simulink model "CDPM"  (R2013a)
settings: Solver=ode45  StartTime=0.0  StopTime=30  RelTol=1e-3
undefined symbols (not defined in the file): A
libraries: fl_lib x52, dspmtrx3 x21, nesl_utility x16, vrlib x12, simulink x9, elec_lib x8, sdl_lib x4, dspsigops x4, elec_controlled_stepper_lib x4
(part 1 of 2)
settings Model: Creator=Anirudh  LastModifiedBy=Anirudh

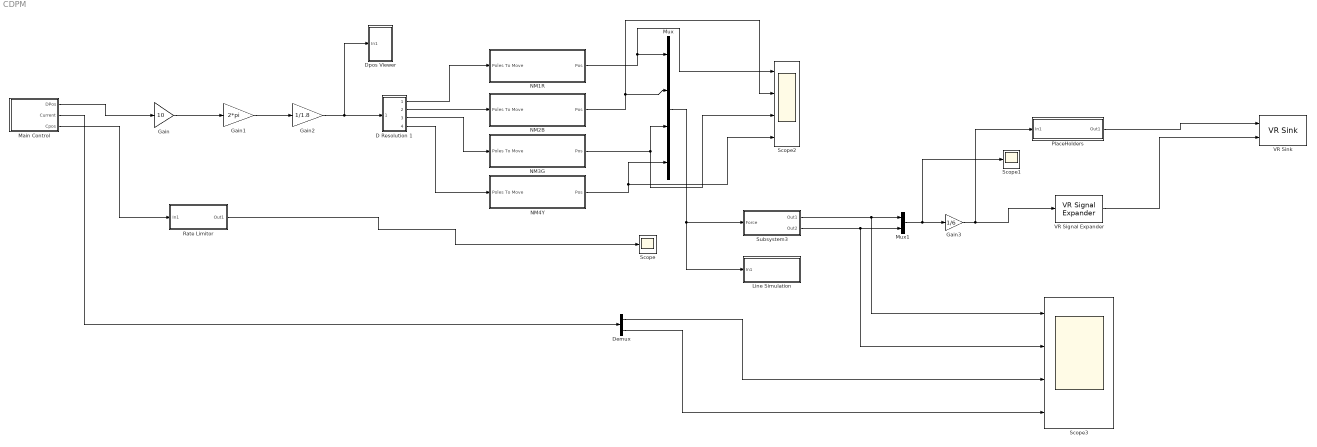
== system CDPM ==
  D Resolution 1 : Subsystem
  Demux : Demux  Outputs=2
  Dpos Viewer : Subsystem
  Gain : Gain  Gain=10
  Gain1 : Gain  Gain=2*pi
  Gain2 : Gain  Gain=1/1.8
  Gain3 : Gain  Gain=1/6
  Line Simulation : Subsystem
  "Main Control " : Subsystem
  Mux : Mux
  Mux1 : Mux  Inputs=2
  "NM1R " : Subsystem
  NM2B : Subsystem
  NM3G : Subsystem
  "NM4Y " : Subsystem
  "PlaceHolders " : Subsystem
  Rate Limitor : Subsystem
  Scope : Scope
      settings: SaveName=ScopeData5
  Scope1 : Scope
      settings: YMin=-3.25  YMax=-1  SaveName=ScopeData7
  Scope2 : Scope  NumInputPorts=4
      settings: TickLabels=on  ShowLegends=on  YMin=-0.79~0.2225~0.309~0.7675  YMax=-0.7675~0.24~0.318~0.79
  Scope3 : Scope  NumInputPorts=4
      settings: YMin=-5~-5~-5~-5  YMax=5~5~5~5  SaveName=ScopeData8
  Subsystem3 : Subsystem
  VR Signal Expander : vrlib/VR Signal Expander  outwidth=3  outidx=[1 3]
  VR Sink : vrlib/VR Sink  InstantiateOnLoad=on  SampleTime=0.1  ViewEnable=on  RemoteChange=off  RemoteView=off  FieldsWritten=LINES.point.3.-1.1.double#EoF.translation.3.1.1.double  WorldFileName=CDPM.wrl  AutoView=on  VideoDimensions=[]  AllowVariableSize=off
  wires:
  "Main Control "/1("DPos ") -> Gain/1
  Gain/1 -> Gain1/1
  Gain1/1 -> Gain2/1
  Gain2/1 -> D Resolution 1/1(In1), Dpos Viewer/1(In1)
  D Resolution 1/1(Out1) -> "NM1R "/1("Poles To Move ")
  "Main Control "/2("Current ") -> Demux/1
  "NM1R "/1(Pos) -> Scope2/1, Mux/1
  D Resolution 1/2(Out2) -> NM2B/1("Poles To Move ")
  D Resolution 1/3(Out3) -> NM3G/1("Poles To Move ")
  D Resolution 1/4(Out4) -> "NM4Y "/1("Poles To Move ")
  "NM4Y "/1(Pos) -> Mux/4, Scope2/4
  NM2B/1(Pos) -> Scope2/2, Mux/2
  NM3G/1(Pos) -> Mux/3, Scope2/3
  Subsystem3/1(Out1) -> Scope3/1, Mux1/1
  Subsystem3/2(Out2) -> Scope3/2, Mux1/2
  "Main Control "/3(Cpos) -> Rate Limitor/1(In1)
  Rate Limitor/1(Out1) -> Scope/1
  Mux1/1 -> Scope1/1, Gain3/1
  Gain3/1 -> "PlaceHolders "/1(In1), VR Signal Expander/1
  Demux/1 -> Scope3/3
  Demux/2 -> Scope3/4
  VR Signal Expander/1 -> VR Sink/2
  "PlaceHolders "/1(Out1) -> VR Sink/1
  Mux/1 -> Line Simulation/1(In1), Subsystem3/1(Force)

== system CDPM/D Resolution 1 ==
  In1 : Inport
  Submatrix : dspmtrx3/Submatrix  RowSpan=All rows  RowStartMode=First  RowStartIndex=1  RowEndMode=Last  RowEndIndex=1  ColSpan=One column  ColStartMode=Index  ColStartIndex=1  ColEndMode=Last  ColEndIndex=1
  Submatrix1 : dspmtrx3/Submatrix  RowSpan=One row  RowStartMode=Index  RowStartIndex=1  RowEndMode=Last  RowEndIndex=1  ColSpan=One column  ColStartMode=Index  ColStartIndex=2  ColEndMode=Last  ColEndIndex=1
  Submatrix2 : dspmtrx3/Submatrix  RowSpan=All rows  RowStartMode=Index  RowStartIndex=2  RowEndMode=Last  RowEndIndex=1  ColSpan=One column  ColStartMode=Index  ColStartIndex=3  ColEndMode=Last  ColEndIndex=1
  Submatrix3 : dspmtrx3/Submatrix  RowSpan=All rows  RowStartMode=Index  RowStartIndex=2  RowEndMode=Last  RowEndIndex=1  ColSpan=One column  ColStartMode=Index  ColStartIndex=4  ColEndMode=Last  ColEndIndex=1
  Out1 : Outport
  Out2 : Outport  Port=2
  Out3 : Outport  Port=3
  Out4 : Outport  Port=4
  wires:
  Submatrix2/1 -> Out3/1
  Submatrix1/1 -> Out2/1
  Submatrix3/1 -> Out4/1
  Submatrix/1 -> Out1/1
  In1/1 -> Submatrix/1, Submatrix1/1, Submatrix2/1, Submatrix3/1

== system CDPM/Dpos Viewer ==
  In1 : Inport
  D Resolution 1 : Subsystem
  Scope1 : Scope  NumInputPorts=4
      settings: TimeRange=5  YMin=-700~-800~-300~-200  YMax=400~700~700~400  SaveName=ScopeData3
  wires:
  D Resolution 1/4(Out4) -> Scope1/4
  D Resolution 1/2(Out2) -> Scope1/2
  D Resolution 1/1(Out1) -> Scope1/1
  In1/1 -> D Resolution 1/1(In1)
  D Resolution 1/3(Out3) -> Scope1/3

== system CDPM/Line Simulation ==
  In1 : Inport
  Demux : Demux
  VR Signal Expander{,1..3} (4 alike) : vrlib/VR Signal Expander  outwidth=4  outidx=[4]
  VR Sink : vrlib/VR Sink  InstantiateOnLoad=on  SampleTime=0.1  ViewEnable=on  RemoteChange=off  RemoteView=off  FieldsWritten=N2YR.rotation.4.1.1.double#N1RR.rotation.4.1.1.double#N3BR.rotation.4.1.1.double#N4GR.rotation.4.1.1.double  WorldFileName=CDPM.wrl  AutoView=off  VideoDimensions=[]  AllowVariableSize=off
  wires:
  VR Signal Expander/1 -> VR Sink/2
  In1/1 -> Demux/1
  Demux/1 -> VR Signal Expander/1
  Demux/2 -> VR Signal Expander1/1
  VR Signal Expander2/1 -> VR Sink/3
  Demux/3 -> VR Signal Expander2/1
  VR Signal Expander3/1 -> VR Sink/4
  Demux/4 -> VR Signal Expander3/1
  VR Signal Expander1/1 -> VR Sink/1

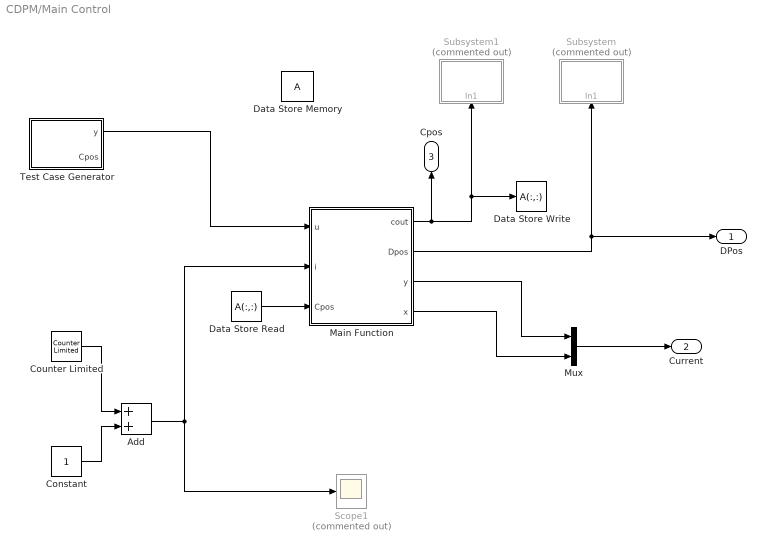
== system CDPM/Main Control  ==
  Add : Sum
  Constant : Constant
  Counter Limited : simulink/Sources/Counter Limited  uplimit=15  tsamp=1
  Data Store Memory : DataStoreMemory  ReadBeforeWriteMsg=warning  WriteAfterWriteMsg=warning  WriteAfterReadMsg=warning  InitialValue=[30,30,30,30]  VectorParams1D=off
  Data Store Read : DataStoreRead  SampleTime=1  DataStoreElements=A(:,:)
  Data Store Write : DataStoreWrite  SampleTime=2  DataStoreElements=A(:,:)
  "Main Function " : MATLAB Function  TreatAsAtomicUnit=on  SystemSampleTime=1
  Mux : Mux  Inputs=2
  Scope1 : Scope  Commented=on
      settings: SaveName=ScopeData6
  Subsystem : Subsystem  Commented=on
  Subsystem1 : Subsystem  Commented=on
  "Test Case Generator " : MATLAB Function
  "DPos " : Outport
  "Current " : Outport  Port=2
  Cpos : Outport  Port=3
  wires:
  Constant/1 -> Add/2
  "Main Function "/2(Dpos) -> "DPos "/1, Subsystem/1(In1)
  Counter Limited/1 -> Add/1
  Add/1 -> "Main Function "/2(i), Scope1/1
  "Main Function "/1(cout) -> Subsystem1/1(In1), Data Store Write/1, Cpos/1
  "Test Case Generator "/1(y) -> "Main Function "/1(u)
  Mux/1 -> "Current "/1
  "Main Function "/3(y) -> Mux/1
  "Main Function "/4(x) -> Mux/2
  Data Store Read/1 -> "Main Function "/3(Cpos)

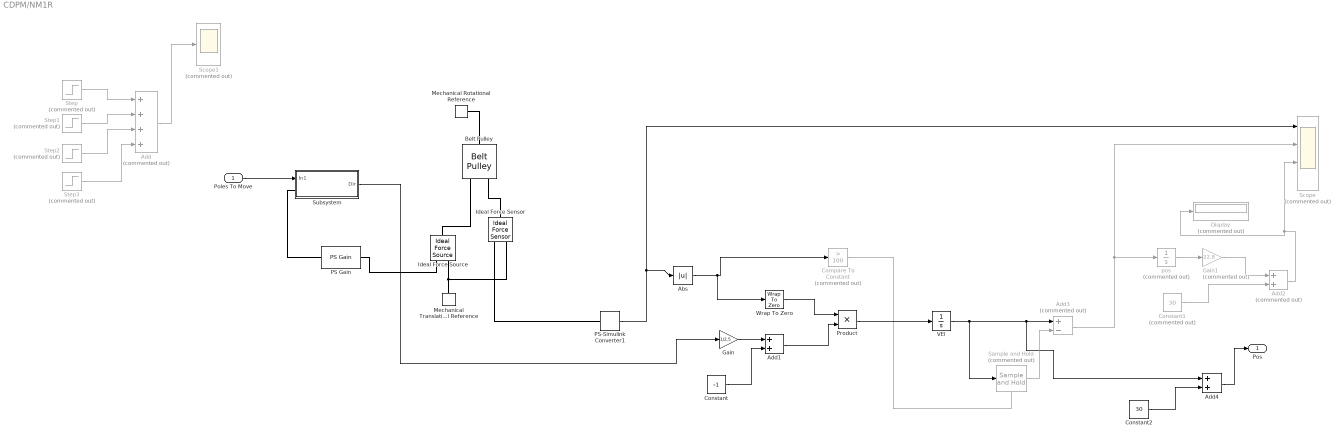
== system CDPM/NM1R  ==
  "Poles To Move " : Inport
  Abs : Abs
  Add : Sum  Commented=on  Inputs=++++
  Add1 : Sum
  Add2 : Sum  Commented=on
  Add3 : Sum  Commented=on  Inputs=+-
  Add4 : Sum
  Belt Pulley : sdl_lib/Couplings & Drives/Belt Pulley  belt_type=1  sheave_ang=30 deg  num_belts=1  linear_density=0.6 kg/m  breakable=0  F_max=1e+5 N  check_tension=0  r_pulley=0.15 m  b_pulley=0.001 N*m/(rad/s)  model_inertia=0  pulley_inertia=0.01 kg*m^2  initial_velocity=0 rad/s  mu=0.5  phi_wrap=180 deg  v_thr=0.001 m/s  LocalVarLogging=[]
  Compare To Constant : simulink/Logic and Bit Operations/Compare To Constant  Commented=on  relop=>  const=100  OutDataTypeStr=uint8
  Constant : Constant  Value=-1
  Constant1 : Constant  Commented=on  Value=30
  Constant2 : Constant  Value=30
  Display : Display  Commented=on
  Gain : Gain  Gain=1/2.5
  Gain1 : Gain  Commented=on  Gain=22.8
  Ideal Force Sensor : fl_lib/Mechanical/Mechanical Sensors/Ideal Force Sensor  v_Log=off  f_Log=off  LocalVarNames=|v|f  LocalVarDescs=|v|f  LocalVarLogging=[0 0]
  Ideal Force Source : fl_lib/Mechanical/Mechanical Sources/Ideal Force Source  v_Log=off  f_Log=off  LocalVarNames=|v|f  LocalVarDescs=|v|f  LocalVarLogging=[0 0]
  Mechanical Rotational Reference : fl_lib/Mechanical/Rotational Elements/Mechanical Rotational Reference  t_Log=off  LocalVarNames=|t  LocalVarDescs=|t  LocalVarLogging=0
  Mechanical Translational Reference : fl_lib/Mechanical/Translational Elements/Mechanical Translational Reference  f_Log=off  LocalVarNames=|f  LocalVarDescs=|f  LocalVarLogging=0
  PS Gain : fl_lib/Physical Signals/Functions/PS Gain  gain=100  LocalVarLogging=[]
  PS-Simulink Converter1 : nesl_utility/PS-Simulink Converter  PhysicalDomain=network_engine_domain  SubClassName=ps_output  LeftPortType=input  RightPortType=output  PseudoPeriodic=off  Frequencies=[]  Unit=N  AffineConversion=off
  Product : Product
  Sample and Hold : dspsigops/Sample and Hold  Commented=on  trig=Either edge  initCond=0  latchinput=off
  Scope : Scope  Commented=on  NumInputPorts=4
      settings: TickLabels=on  YMin=-5~-5~-5~-5  YMax=5~5~5~5  SaveName=ScopeData4
  Scope1 : Scope  Commented=on
  Step : Step  Commented=on  Time=5  After=10  SampleTime=0
  Step1 : Step  Commented=on  Time=10  After=10  SampleTime=0
  Step2 : Step  Commented=on  Time=15  After=-10  SampleTime=0
  Step3 : Step  Commented=on  Time=20  After=-10  SampleTime=0
  Subsystem : Subsystem
  VEl : Integrator
  Wrap To Zero : simulink/Discontinuities/Wrap To Zero  Threshold=50
  pos : Integrator  Commented=on
  Pos : Outport
  wires:
  Add/1 -> Scope1/1
  Step/1 -> Add/1
  Step1/1 -> Add/2
  Step2/1 -> Add/3
  Step3/1 -> Add/4
  "Poles To Move "/1 -> Subsystem/1(In1)
  Subsystem/1("Dir ") -> Gain/1
  Gain/1 -> Add1/1
  Constant/1 -> Add1/2
  Add1/1 -> Product/2
  Abs/1 -> Wrap To Zero/1, Compare To Constant/1
  Constant1/1 -> Add2/2
  pos/1 -> Gain1/1
  Gain1/1 -> Add2/1
  VEl/1 -> Sample and Hold/1, Add4/1, Add3/1
  Sample and Hold/1 -> Add3/2
  Add3/1 -> pos/1, Scope/2
  Add2/1 -> Scope/3, Display/1
  PS-Simulink Converter1/1 -> Scope/1, Abs/1
  Compare To Constant/1 -> Sample and Hold/Trigger
  Wrap To Zero/1 -> Product/1
  Constant2/1 -> Add4/2
  Add4/1 -> Pos/1
  Product/1 -> VEl/1
  connections:
  Ideal Force Source/RConn2 -- Ideal Force Sensor/RConn1 -- Mechanical Translational Reference/LConn1
  PS Gain/RConn1 -- Ideal Force Source/RConn1
  Belt Pulley/RConn2 -- Ideal Force Source/LConn1
  Subsystem/LConn1 -- PS Gain/LConn1
  Belt Pulley/RConn1 -- Ideal Force Sensor/LConn1
  PS-Simulink Converter1/LConn1 -- Ideal Force Sensor/RConn2
  Mechanical Rotational Reference/LConn1 -- Belt Pulley/LConn1

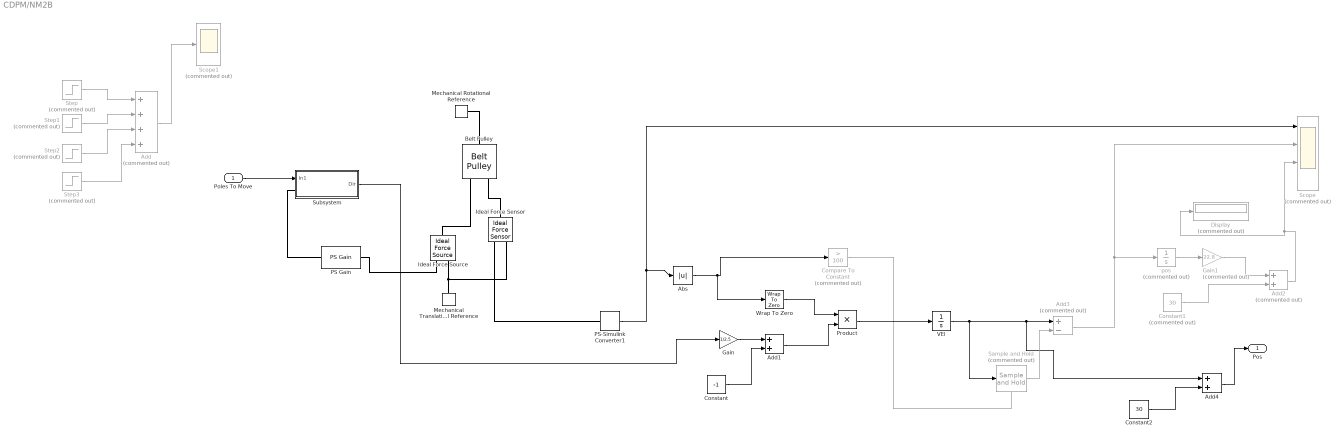
== system CDPM/NM2B ==
  "Poles To Move " : Inport
  Abs : Abs
  Add : Sum  Commented=on  Inputs=++++
  Add1 : Sum
  Add2 : Sum  Commented=on
  Add3 : Sum  Commented=on  Inputs=+-
  Add4 : Sum
  Belt Pulley : sdl_lib/Couplings & Drives/Belt Pulley  belt_type=1  sheave_ang=30 deg  num_belts=1  linear_density=0.6 kg/m  breakable=0  F_max=1e+5 N  check_tension=0  r_pulley=0.15 m  b_pulley=0.001 N*m/(rad/s)  model_inertia=0  pulley_inertia=0.01 kg*m^2  initial_velocity=0 rad/s  mu=0.5  phi_wrap=180 deg  v_thr=0.001 m/s  LocalVarLogging=[]
  Compare To Constant : simulink/Logic and Bit Operations/Compare To Constant  Commented=on  relop=>  const=100  OutDataTypeStr=uint8
  Constant : Constant  Value=-1
  Constant1 : Constant  Commented=on  Value=30
  Constant2 : Constant  Value=30
  Display : Display  Commented=on
  Gain : Gain  Gain=1/2.5
  Gain1 : Gain  Commented=on  Gain=22.8
  Ideal Force Sensor : fl_lib/Mechanical/Mechanical Sensors/Ideal Force Sensor  v_Log=off  f_Log=off  LocalVarNames=|v|f  LocalVarDescs=|v|f  LocalVarLogging=[0 0]
  Ideal Force Source : fl_lib/Mechanical/Mechanical Sources/Ideal Force Source  v_Log=off  f_Log=off  LocalVarNames=|v|f  LocalVarDescs=|v|f  LocalVarLogging=[0 0]
  Mechanical Rotational Reference : fl_lib/Mechanical/Rotational Elements/Mechanical Rotational Reference  t_Log=off  LocalVarNames=|t  LocalVarDescs=|t  LocalVarLogging=0
  Mechanical Translational Reference : fl_lib/Mechanical/Translational Elements/Mechanical Translational Reference  f_Log=off  LocalVarNames=|f  LocalVarDescs=|f  LocalVarLogging=0
  PS Gain : fl_lib/Physical Signals/Functions/PS Gain  gain=100  LocalVarLogging=[]
  PS-Simulink Converter1 : nesl_utility/PS-Simulink Converter  PhysicalDomain=network_engine_domain  SubClassName=ps_output  LeftPortType=input  RightPortType=output  PseudoPeriodic=off  Frequencies=[]  Unit=N  AffineConversion=off
  Product : Product
  Sample and Hold : dspsigops/Sample and Hold  Commented=on  trig=Either edge  initCond=0  latchinput=off
  Scope : Scope  Commented=on  NumInputPorts=4
      settings: TickLabels=on  YMin=-5~-5~-5~-5  YMax=5~5~5~5  SaveName=ScopeData4
  Scope1 : Scope  Commented=on
  Step : Step  Commented=on  Time=5  After=10  SampleTime=0
  Step1 : Step  Commented=on  Time=10  After=10  SampleTime=0
  Step2 : Step  Commented=on  Time=15  After=-10  SampleTime=0
  Step3 : Step  Commented=on  Time=20  After=-10  SampleTime=0
  Subsystem : Subsystem
  VEl : Integrator
  Wrap To Zero : simulink/Discontinuities/Wrap To Zero  Threshold=50
  pos : Integrator  Commented=on
  Pos : Outport
  wires:
  Add/1 -> Scope1/1
  Step/1 -> Add/1
  Step1/1 -> Add/2
  Step2/1 -> Add/3
  Step3/1 -> Add/4
  "Poles To Move "/1 -> Subsystem/1(In1)
  Subsystem/1("Dir ") -> Gain/1
  Gain/1 -> Add1/1
  Constant/1 -> Add1/2
  Add1/1 -> Product/2
  Abs/1 -> Wrap To Zero/1, Compare To Constant/1
  Constant1/1 -> Add2/2
  pos/1 -> Gain1/1
  Gain1/1 -> Add2/1
  VEl/1 -> Sample and Hold/1, Add4/1, Add3/1
  Sample and Hold/1 -> Add3/2
  Add3/1 -> pos/1, Scope/2
  Add2/1 -> Scope/3, Display/1
  PS-Simulink Converter1/1 -> Scope/1, Abs/1
  Compare To Constant/1 -> Sample and Hold/Trigger
  Wrap To Zero/1 -> Product/1
  Constant2/1 -> Add4/2
  Add4/1 -> Pos/1
  Product/1 -> VEl/1
  connections:
  Ideal Force Source/RConn2 -- Ideal Force Sensor/RConn1 -- Mechanical Translational Reference/LConn1
  PS Gain/RConn1 -- Ideal Force Source/RConn1
  Belt Pulley/RConn2 -- Ideal Force Source/LConn1
  Subsystem/LConn1 -- PS Gain/LConn1
  Belt Pulley/RConn1 -- Ideal Force Sensor/LConn1
  PS-Simulink Converter1/LConn1 -- Ideal Force Sensor/RConn2
  Mechanical Rotational Reference/LConn1 -- Belt Pulley/LConn1

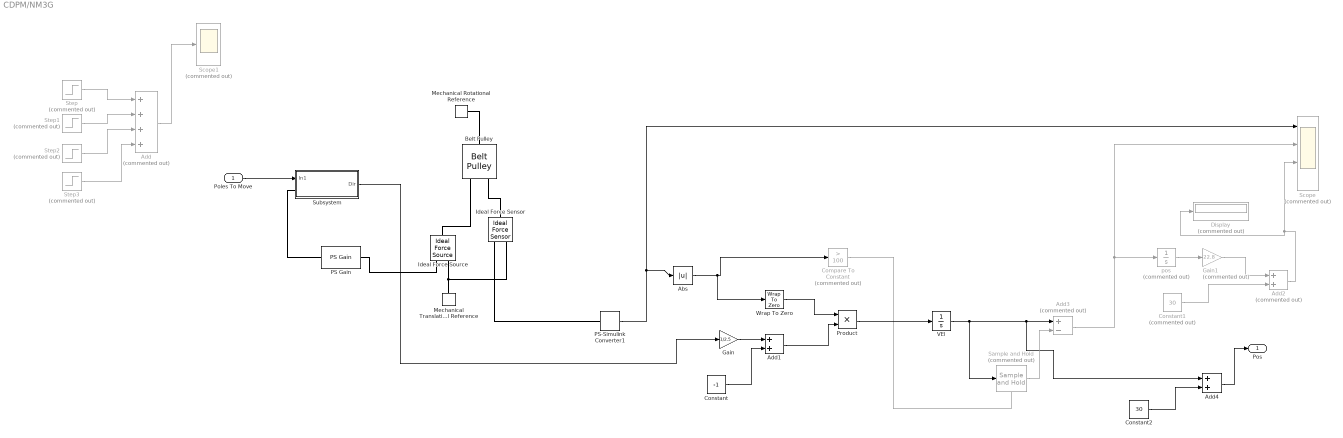
== system CDPM/NM3G ==
  "Poles To Move " : Inport
  Abs : Abs
  Add : Sum  Commented=on  Inputs=++++
  Add1 : Sum
  Add2 : Sum  Commented=on
  Add3 : Sum  Commented=on  Inputs=+-
  Add4 : Sum
  Belt Pulley : sdl_lib/Couplings & Drives/Belt Pulley  belt_type=1  sheave_ang=30 deg  num_belts=1  linear_density=0.6 kg/m  breakable=0  F_max=1e+5 N  check_tension=0  r_pulley=0.15 m  b_pulley=0.001 N*m/(rad/s)  model_inertia=0  pulley_inertia=0.01 kg*m^2  initial_velocity=0 rad/s  mu=0.5  phi_wrap=180 deg  v_thr=0.001 m/s  LocalVarLogging=[]
  Compare To Constant : simulink/Logic and Bit Operations/Compare To Constant  Commented=on  relop=>  const=100  OutDataTypeStr=uint8
  Constant : Constant  Value=-1
  Constant1 : Constant  Commented=on  Value=30
  Constant2 : Constant  Value=30
  Display : Display  Commented=on
  Gain : Gain  Gain=1/2.5
  Gain1 : Gain  Commented=on  Gain=22.8
  Ideal Force Sensor : fl_lib/Mechanical/Mechanical Sensors/Ideal Force Sensor  v_Log=off  f_Log=off  LocalVarNames=|v|f  LocalVarDescs=|v|f  LocalVarLogging=[0 0]
  Ideal Force Source : fl_lib/Mechanical/Mechanical Sources/Ideal Force Source  v_Log=off  f_Log=off  LocalVarNames=|v|f  LocalVarDescs=|v|f  LocalVarLogging=[0 0]
  Mechanical Rotational Reference : fl_lib/Mechanical/Rotational Elements/Mechanical Rotational Reference  t_Log=off  LocalVarNames=|t  LocalVarDescs=|t  LocalVarLogging=0
  Mechanical Translational Reference : fl_lib/Mechanical/Translational Elements/Mechanical Translational Reference  f_Log=off  LocalVarNames=|f  LocalVarDescs=|f  LocalVarLogging=0
  PS Gain : fl_lib/Physical Signals/Functions/PS Gain  gain=100  LocalVarLogging=[]
  PS-Simulink Converter1 : nesl_utility/PS-Simulink Converter  PhysicalDomain=network_engine_domain  SubClassName=ps_output  LeftPortType=input  RightPortType=output  PseudoPeriodic=off  Frequencies=[]  Unit=N  AffineConversion=off
  Product : Product
  Sample and Hold : dspsigops/Sample and Hold  Commented=on  trig=Either edge  initCond=0  latchinput=off
  Scope : Scope  Commented=on  NumInputPorts=4
      settings: TickLabels=on  YMin=-5~-5~-5~-5  YMax=5~5~5~5  SaveName=ScopeData4
  Scope1 : Scope  Commented=on
  Step : Step  Commented=on  Time=5  After=10  SampleTime=0
  Step1 : Step  Commented=on  Time=10  After=10  SampleTime=0
  Step2 : Step  Commented=on  Time=15  After=-10  SampleTime=0
  Step3 : Step  Commented=on  Time=20  After=-10  SampleTime=0
  Subsystem : Subsystem
  VEl : Integrator
  Wrap To Zero : simulink/Discontinuities/Wrap To Zero  Threshold=50
  pos : Integrator  Commented=on
  Pos : Outport
  wires:
  Add/1 -> Scope1/1
  Step/1 -> Add/1
  Step1/1 -> Add/2
  Step2/1 -> Add/3
  Step3/1 -> Add/4
  "Poles To Move "/1 -> Subsystem/1(In1)
  Subsystem/1("Dir ") -> Gain/1
  Gain/1 -> Add1/1
  Constant/1 -> Add1/2
  Add1/1 -> Product/2
  Abs/1 -> Wrap To Zero/1, Compare To Constant/1
  Constant1/1 -> Add2/2
  pos/1 -> Gain1/1
  Gain1/1 -> Add2/1
  VEl/1 -> Sample and Hold/1, Add4/1, Add3/1
  Sample and Hold/1 -> Add3/2
  Add3/1 -> pos/1, Scope/2
  Add2/1 -> Scope/3, Display/1
  PS-Simulink Converter1/1 -> Scope/1, Abs/1
  Compare To Constant/1 -> Sample and Hold/Trigger
  Wrap To Zero/1 -> Product/1
  Constant2/1 -> Add4/2
  Add4/1 -> Pos/1
  Product/1 -> VEl/1
  connections:
  Ideal Force Source/RConn2 -- Ideal Force Sensor/RConn1 -- Mechanical Translational Reference/LConn1
  PS Gain/RConn1 -- Ideal Force Source/RConn1
  Belt Pulley/RConn2 -- Ideal Force Source/LConn1
  Subsystem/LConn1 -- PS Gain/LConn1
  Belt Pulley/RConn1 -- Ideal Force Sensor/LConn1
  PS-Simulink Converter1/LConn1 -- Ideal Force Sensor/RConn2
  Mechanical Rotational Reference/LConn1 -- Belt Pulley/LConn1

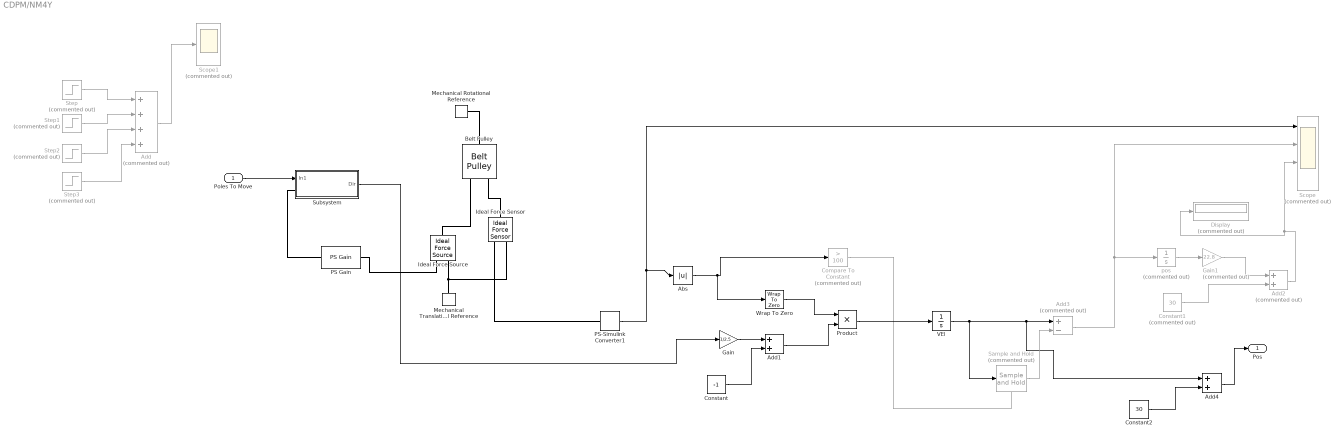
== system CDPM/NM4Y  ==
  "Poles To Move " : Inport
  Abs : Abs
  Add : Sum  Commented=on  Inputs=++++
  Add1 : Sum
  Add2 : Sum  Commented=on
  Add3 : Sum  Commented=on  Inputs=+-
  Add4 : Sum
  Belt Pulley : sdl_lib/Couplings & Drives/Belt Pulley  belt_type=1  sheave_ang=30 deg  num_belts=1  linear_density=0.6 kg/m  breakable=0  F_max=1e+5 N  check_tension=0  r_pulley=0.15 m  b_pulley=0.001 N*m/(rad/s)  model_inertia=0  pulley_inertia=0.01 kg*m^2  initial_velocity=0 rad/s  mu=0.5  phi_wrap=180 deg  v_thr=0.001 m/s  LocalVarLogging=[]
  Compare To Constant : simulink/Logic and Bit Operations/Compare To Constant  Commented=on  relop=>  const=100  OutDataTypeStr=uint8
  Constant : Constant  Value=-1
  Constant1 : Constant  Commented=on  Value=30
  Constant2 : Constant  Value=30
  Display : Display  Commented=on
  Gain : Gain  Gain=1/2.5
  Gain1 : Gain  Commented=on  Gain=22.8
  Ideal Force Sensor : fl_lib/Mechanical/Mechanical Sensors/Ideal Force Sensor  v_Log=off  f_Log=off  LocalVarNames=|v|f  LocalVarDescs=|v|f  LocalVarLogging=[0 0]
  Ideal Force Source : fl_lib/Mechanical/Mechanical Sources/Ideal Force Source  v_Log=off  f_Log=off  LocalVarNames=|v|f  LocalVarDescs=|v|f  LocalVarLogging=[0 0]
  Mechanical Rotational Reference : fl_lib/Mechanical/Rotational Elements/Mechanical Rotational Reference  t_Log=off  LocalVarNames=|t  LocalVarDescs=|t  LocalVarLogging=0
  Mechanical Translational Reference : fl_lib/Mechanical/Translational Elements/Mechanical Translational Reference  f_Log=off  LocalVarNames=|f  LocalVarDescs=|f  LocalVarLogging=0
  PS Gain : fl_lib/Physical Signals/Functions/PS Gain  gain=100  LocalVarLogging=[]
  PS-Simulink Converter1 : nesl_utility/PS-Simulink Converter  PhysicalDomain=network_engine_domain  SubClassName=ps_output  LeftPortType=input  RightPortType=output  PseudoPeriodic=off  Frequencies=[]  Unit=N  AffineConversion=off
  Product : Product
  Sample and Hold : dspsigops/Sample and Hold  Commented=on  trig=Either edge  initCond=0  latchinput=off
  Scope : Scope  Commented=on  NumInputPorts=4
      settings: TickLabels=on  YMin=-5~-5~-5~-5  YMax=5~5~5~5  SaveName=ScopeData4
  Scope1 : Scope  Commented=on
  Step : Step  Commented=on  Time=5  After=10  SampleTime=0
  Step1 : Step  Commented=on  Time=10  After=10  SampleTime=0
  Step2 : Step  Commented=on  Time=15  After=-10  SampleTime=0
  Step3 : Step  Commented=on  Time=20  After=-10  SampleTime=0
  Subsystem : Subsystem
  VEl : Integrator
  Wrap To Zero : simulink/Discontinuities/Wrap To Zero  Threshold=50
  pos : Integrator  Commented=on
  Pos : Outport
  wires:
  Add/1 -> Scope1/1
  Step/1 -> Add/1
  Step1/1 -> Add/2
  Step2/1 -> Add/3
  Step3/1 -> Add/4
  "Poles To Move "/1 -> Subsystem/1(In1)
  Subsystem/1("Dir ") -> Gain/1
  Gain/1 -> Add1/1
  Constant/1 -> Add1/2
  Add1/1 -> Product/2
  Abs/1 -> Wrap To Zero/1, Compare To Constant/1
  Constant1/1 -> Add2/2
  pos/1 -> Gain1/1
  Gain1/1 -> Add2/1
  VEl/1 -> Sample and Hold/1, Add4/1, Add3/1
  Sample and Hold/1 -> Add3/2
  Add3/1 -> pos/1, Scope/2
  Add2/1 -> Scope/3, Display/1
  PS-Simulink Converter1/1 -> Scope/1, Abs/1
  Compare To Constant/1 -> Sample and Hold/Trigger
  Wrap To Zero/1 -> Product/1
  Constant2/1 -> Add4/2
  Add4/1 -> Pos/1
  Product/1 -> VEl/1
  connections:
  Ideal Force Source/RConn2 -- Ideal Force Sensor/RConn1 -- Mechanical Translational Reference/LConn1
  PS Gain/RConn1 -- Ideal Force Source/RConn1
  Belt Pulley/RConn2 -- Ideal Force Source/LConn1
  Subsystem/LConn1 -- PS Gain/LConn1
  Belt Pulley/RConn1 -- Ideal Force Sensor/LConn1
  PS-Simulink Converter1/LConn1 -- Ideal Force Sensor/RConn2
  Mechanical Rotational Reference/LConn1 -- Belt Pulley/LConn1

== system CDPM/PlaceHolders  ==
  In1 : Inport
  Matrix Concatenate : Concatenate  NumInputs=5  Mode=Multidimensional array
  Transpose{,1..4} (5 alike) : dspmtrx3/Transpose  Hermitian=off  overflowFlag=off
  VR Placeholder{,1..3} (4 alike) : vrlib/VR Placeholder  outwidth=3
  VR Signal Expander1 : vrlib/VR Signal Expander  outwidth=3  outidx=[1 3]
  Out1 : Outport
  wires:
  VR Placeholder2/1 -> Transpose3/1
  Transpose3/1 -> Matrix Concatenate/4
  Transpose1/1 -> Matrix Concatenate/2
  Transpose2/1 -> Matrix Concatenate/3
  Matrix Concatenate/1 -> Out1/1
  Transpose4/1 -> Matrix Concatenate/5
  VR Placeholder/1 -> Transpose1/1
  VR Placeholder3/1 -> Transpose4/1
  VR Signal Expander1/1 -> Transpose/1
  VR Placeholder1/1 -> Transpose2/1
  Transpose/1 -> Matrix Concatenate/1
  In1/1 -> VR Signal Expander1/1

== system CDPM/Rate Limitor ==
  In1 : Inport
  Demux : Demux
  Mux : Mux
  Rate Limiter{,1..3} (4 alike) : RateLimiter  RisingSlewLimit=25  FallingSlewLimit=-25
  Out1 : Outport
  wires:
  In1/1 -> Demux/1
  Demux/1 -> Rate Limiter/1
  Demux/2 -> Rate Limiter1/1
  Demux/3 -> Rate Limiter2/1
  Demux/4 -> Rate Limiter3/1
  Rate Limiter3/1 -> Mux/4
  Rate Limiter/1 -> Mux/1
  Rate Limiter2/1 -> Mux/3
  Rate Limiter1/1 -> Mux/2
  Mux/1 -> Out1/1

== system CDPM/Subsystem3 ==
  Force : Inport
  Constant : Constant  Value=40
  Demux1 : Demux
  Herons Formula : Subsystem
  Herons Formula1 : Subsystem
  Out1 : Outport
  Out2 : Outport  Port=2
  wires:
  Force/1 -> Demux1/1
  Demux1/1 -> Herons Formula/1(In1)
  Demux1/2 -> Herons Formula1/1(In1), Herons Formula/2(In2)
  Constant/1 -> Herons Formula/3(In3), Herons Formula1/3(In3)
  Herons Formula/1(Out1) -> Out1/1
  Herons Formula1/1(Out1) -> Out2/1
  Demux1/4 -> Herons Formula1/2(In2)

== system CDPM/Dpos Viewer/D Resolution 1 ==
  In1 : Inport
  Submatrix : dspmtrx3/Submatrix  RowSpan=All rows  RowStartMode=First  RowStartIndex=1  RowEndMode=Last  RowEndIndex=1  ColSpan=One column  ColStartMode=Index  ColStartIndex=1  ColEndMode=Last  ColEndIndex=1
  Submatrix1 : dspmtrx3/Submatrix  RowSpan=One row  RowStartMode=Index  RowStartIndex=1  RowEndMode=Last  RowEndIndex=1  ColSpan=One column  ColStartMode=Index  ColStartIndex=2  ColEndMode=Last  ColEndIndex=1
  Submatrix2 : dspmtrx3/Submatrix  RowSpan=All rows  RowStartMode=Index  RowStartIndex=2  RowEndMode=Last  RowEndIndex=1  ColSpan=One column  ColStartMode=Index  ColStartIndex=3  ColEndMode=Last  ColEndIndex=1
  Submatrix3 : dspmtrx3/Submatrix  RowSpan=All rows  RowStartMode=Index  RowStartIndex=2  RowEndMode=Last  RowEndIndex=1  ColSpan=One column  ColStartMode=Index  ColStartIndex=4  ColEndMode=Last  ColEndIndex=1
  Out1 : Outport
  Out2 : Outport  Port=2
  Out3 : Outport  Port=3
  Out4 : Outport  Port=4
  wires:
  Submatrix2/1 -> Out3/1
  Submatrix1/1 -> Out2/1
  Submatrix3/1 -> Out4/1
  Submatrix/1 -> Out1/1
  In1/1 -> Submatrix/1, Submatrix1/1, Submatrix2/1, Submatrix3/1

== system CDPM/Main Control /Subsystem ==
  In1 : Inport
  "D Resolution " : Subsystem
  Scope : Scope  NumInputPorts=4
      settings: YMin=-5~-5~-5~-5  YMax=5~5~5~5  SaveName=ScopeData2
  wires:
  In1/1 -> "D Resolution "/1(In1)
  "D Resolution "/3(Out3) -> Scope/3
  "D Resolution "/2(Out2) -> Scope/2
  "D Resolution "/4(Out4) -> Scope/4
  "D Resolution "/1(Out1) -> Scope/1

== system CDPM/Main Control /Subsystem1 ==
  In1 : Inport
  D Resolution 1 : Subsystem
  Display : Display
  Scope1 : Scope  NumInputPorts=4
      settings: YMin=-5~-5~-5~-5  YMax=5~5~5~5  SaveName=ScopeData3
  wires:
  D Resolution 1/4(Out4) -> Scope1/4
  D Resolution 1/2(Out2) -> Scope1/2
  D Resolution 1/1(Out1) -> Display/1, Scope1/1
  In1/1 -> D Resolution 1/1(In1)
  D Resolution 1/3(Out3) -> Scope1/3

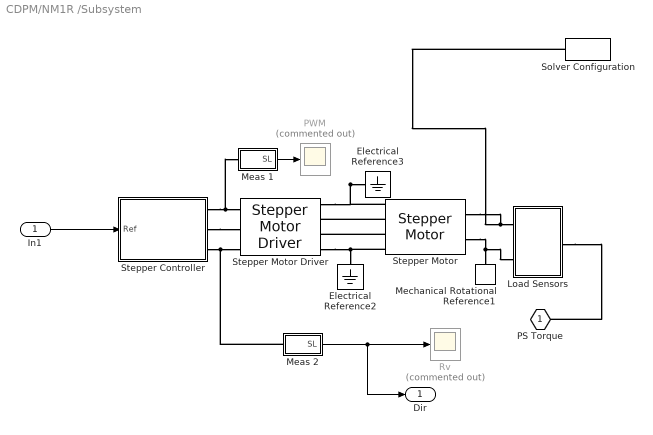
== system CDPM/NM1R /Subsystem ==
  In1 : Inport
  Electrical Reference2 : fl_lib/Electrical/Electrical Elements/Electrical Reference  i_Log=off  LocalVarNames=|i  LocalVarDescs=|i  LocalVarLogging=[]
  Electrical Reference3 : fl_lib/Electrical/Electrical Elements/Electrical Reference  i_Log=off  LocalVarNames=|i  LocalVarDescs=|i  LocalVarLogging=[]
  Load Sensors : Subsystem
  Meas 1 : Subsystem
  Meas 2 : Subsystem
  Mechanical Rotational Reference1 : fl_lib/Mechanical/Rotational Elements/Mechanical Rotational Reference  t_Log=off  LocalVarNames=|t  LocalVarDescs=|t  LocalVarLogging=[]
  PWM : Scope  Commented=on
      settings: TimeRange=2  YMin=-1  YMax=6  SaveName=RPM  SampleTime=0.1
  Rv : Scope  Commented=on
      settings: TimeRange=2  YMin=-1  YMax=6  SaveName=RPM1  SampleTime=0.1
  Solver Configuration : nesl_utility/Solver Configuration  PhysicalDomain=network_engine_domain  SubClassName=solver  LeftPortType=input  RightPortType=generic  Accelerate=off  Tones=[]  Harmonics=[]  SimulateNoise=off  Profile=off  UseLocalSampling=off  EnableSwitchedLinearOptims=on  FrequencyDomain=off  UseCCode=off  UseNewInitialization=off  DoDC=off  ResidualTolerance=1e-9  UseLocalSolver=off  LocalSolverChoice=NE_BACKWARD_EULER_ADVANCER  LocalSolverSampleTime=.001  DoFixedCost=off  MaxNonlinIter=3  MaxModeIter=2  LinearAlgebra=Sparse  DelaysMemoryBudget=1024
  Stepper Controller : Subsystem  BlockChoice=Position Controller
      link override Position Controller/Control algorithm implemented on a microprocessor or dedicated discrete chip/Logic2Volts1: Gain=5
      link override Position Controller/Control algorithm implemented on a microprocessor or dedicated discrete chip/Logic2Volts2: Gain=5
      link override Position Controller/Control algorithm implemented on a microprocessor or dedicated discrete chip/Pulse Generator: f=5000
      settings: AttributesFormatString=%<BlockChoice>  MemberBlocks=Position Controller,Speed Controller
      settings: TemplateBlock=|
      | elec_controlled_stepper_lib/Configurable
      | Subsystem
  Stepper Motor : elec_lib/Actuators & Drivers/Rotational Actuators/Stepper Motor  Ra=1.04 Ohm  La=2.2 mH  Km=0.14 N*m/A  Rm=Inf Ohm  Step=1.8 deg  J=4.5e-5 kg*m^2  B=8e-4 N*m/(rad/s)  speed0=0 rpm  theta0=0 deg  LocalVarLogging=[]  alpha=[ 0.00393 0.00393 ] 1/K  Tmeas=25 C  thermal_masses=[ 100 100 ] J/K  initial_temperatures=[ 25 25 ] C  rotor_thermal_mass=50 J/K  rotor_initial_temperature=25 C  Rm_percent_rotor=90
  Stepper Motor Driver : elec_lib/Actuators & Drivers/Drivers/Stepper Motor Driver  Venable=2.5 V  Vreverse=2.5 V  Vm=24 V  LocalVarLogging=[]
  PS Torque : PMIOPort  Port=1  Side=Left
  "Dir " : Outport
  wires:
  Meas 1/1(SL) -> PWM/1
  In1/1 -> Stepper Controller/1(Ref)
  Meas 2/1(SL) -> "Dir "/1, Rv/1
  connections:
  Electrical Reference3/LConn1 -- Stepper Motor/LConn1 -- Stepper Motor Driver/RConn1
  Electrical Reference2/LConn1 -- Stepper Motor/LConn4 -- Stepper Motor Driver/RConn4
  Load Sensors/LConn1 -- Solver Configuration/RConn1 -- Stepper Motor/RConn1
  Mechanical Rotational Reference1/LConn1 -- Stepper Motor/RConn2 -- Load Sensors/LConn2
  Stepper Motor Driver/LConn1 -- Stepper Controller/RConn1 -- Meas 1/LConn1
  Stepper Controller/RConn2 -- Stepper Motor Driver/LConn2
  Stepper Motor/LConn2 -- Stepper Motor Driver/RConn2
  Stepper Motor/LConn3 -- Stepper Motor Driver/RConn3
  Stepper Controller/RConn3 -- Meas 2/LConn1 -- Stepper Motor Driver/LConn3
  Load Sensors/RConn1 -- PS Torque/RConn1

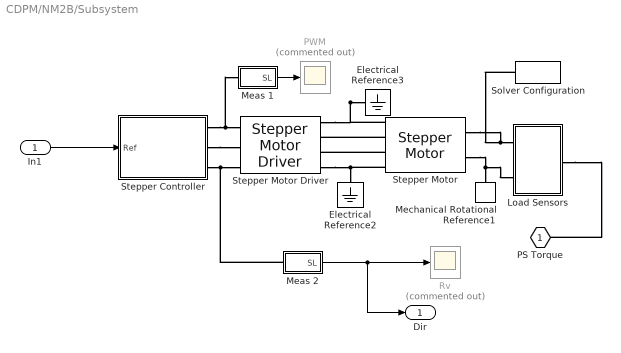
== system CDPM/NM2B/Subsystem ==
  In1 : Inport
  Electrical Reference2 : fl_lib/Electrical/Electrical Elements/Electrical Reference  i_Log=off  LocalVarNames=|i  LocalVarDescs=|i  LocalVarLogging=[]
  Electrical Reference3 : fl_lib/Electrical/Electrical Elements/Electrical Reference  i_Log=off  LocalVarNames=|i  LocalVarDescs=|i  LocalVarLogging=[]
  Load Sensors : Subsystem
  Meas 1 : Subsystem
  Meas 2 : Subsystem
  Mechanical Rotational Reference1 : fl_lib/Mechanical/Rotational Elements/Mechanical Rotational Reference  t_Log=off  LocalVarNames=|t  LocalVarDescs=|t  LocalVarLogging=[]
  PWM : Scope  Commented=on
      settings: TimeRange=2  YMin=-1  YMax=6  SaveName=RPM  SampleTime=0.1
  Rv : Scope  Commented=on
      settings: TimeRange=2  YMin=-1  YMax=6  SaveName=RPM1  SampleTime=0.1
  Solver Configuration : nesl_utility/Solver Configuration  PhysicalDomain=network_engine_domain  SubClassName=solver  LeftPortType=input  RightPortType=generic  Accelerate=off  Tones=[]  Harmonics=[]  SimulateNoise=off  Profile=off  UseLocalSampling=off  EnableSwitchedLinearOptims=on  FrequencyDomain=off  UseCCode=off  UseNewInitialization=off  DoDC=off  ResidualTolerance=1e-9  UseLocalSolver=off  LocalSolverChoice=NE_BACKWARD_EULER_ADVANCER  LocalSolverSampleTime=.001  DoFixedCost=off  MaxNonlinIter=3  MaxModeIter=2  LinearAlgebra=Sparse  DelaysMemoryBudget=1024
  Stepper Controller : Subsystem  BlockChoice=Position Controller
      link override Position Controller/Control algorithm implemented on a microprocessor or dedicated discrete chip/Logic2Volts1: Gain=5
      link override Position Controller/Control algorithm implemented on a microprocessor or dedicated discrete chip/Logic2Volts2: Gain=5
      link override Position Controller/Control algorithm implemented on a microprocessor or dedicated discrete chip/Pulse Generator: f=5000
      settings: AttributesFormatString=%<BlockChoice>  MemberBlocks=Position Controller,Speed Controller
      settings: TemplateBlock=|
      | elec_controlled_stepper_lib/Configurable
      | Subsystem
  Stepper Motor : elec_lib/Actuators & Drivers/Rotational Actuators/Stepper Motor  Ra=1.04 Ohm  La=2.2 mH  Km=0.14 N*m/A  Rm=Inf Ohm  Step=1.8 deg  J=4.5e-5 kg*m^2  B=8e-4 N*m/(rad/s)  speed0=0 rpm  theta0=0 deg  LocalVarLogging=[]  alpha=[ 0.00393 0.00393 ] 1/K  Tmeas=25 C  thermal_masses=[ 100 100 ] J/K  initial_temperatures=[ 25 25 ] C  rotor_thermal_mass=50 J/K  rotor_initial_temperature=25 C  Rm_percent_rotor=90
  Stepper Motor Driver : elec_lib/Actuators & Drivers/Drivers/Stepper Motor Driver  Venable=2.5 V  Vreverse=2.5 V  Vm=24 V  LocalVarLogging=[]
  PS Torque : PMIOPort  Port=1  Side=Left
  "Dir " : Outport
  wires:
  Meas 1/1(SL) -> PWM/1
  In1/1 -> Stepper Controller/1(Ref)
  Meas 2/1(SL) -> "Dir "/1, Rv/1
  connections:
  Electrical Reference3/LConn1 -- Stepper Motor/LConn1 -- Stepper Motor Driver/RConn1
  Electrical Reference2/LConn1 -- Stepper Motor/LConn4 -- Stepper Motor Driver/RConn4
  Load Sensors/LConn1 -- Stepper Motor/RConn1 -- Solver Configuration/RConn1
  Mechanical Rotational Reference1/LConn1 -- Stepper Motor/RConn2 -- Load Sensors/LConn2
  Stepper Motor Driver/LConn1 -- Stepper Controller/RConn1 -- Meas 1/LConn1
  Stepper Controller/RConn2 -- Stepper Motor Driver/LConn2
  Stepper Motor/LConn2 -- Stepper Motor Driver/RConn2
  Stepper Motor/LConn3 -- Stepper Motor Driver/RConn3
  Stepper Controller/RConn3 -- Meas 2/LConn1 -- Stepper Motor Driver/LConn3
  Load Sensors/RConn1 -- PS Torque/RConn1

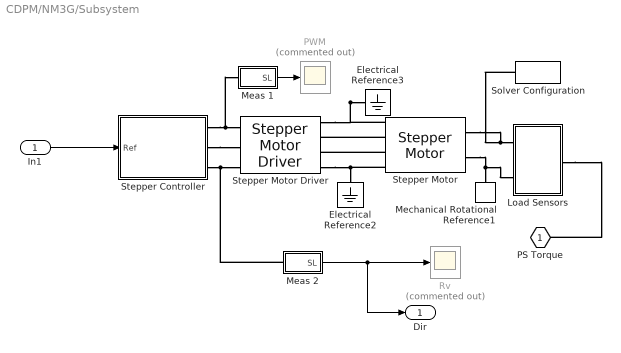
== system CDPM/NM3G/Subsystem ==
  In1 : Inport
  Electrical Reference2 : fl_lib/Electrical/Electrical Elements/Electrical Reference  i_Log=off  LocalVarNames=|i  LocalVarDescs=|i  LocalVarLogging=[]
  Electrical Reference3 : fl_lib/Electrical/Electrical Elements/Electrical Reference  i_Log=off  LocalVarNames=|i  LocalVarDescs=|i  LocalVarLogging=[]
  Load Sensors : Subsystem
  Meas 1 : Subsystem
  Meas 2 : Subsystem
  Mechanical Rotational Reference1 : fl_lib/Mechanical/Rotational Elements/Mechanical Rotational Reference  t_Log=off  LocalVarNames=|t  LocalVarDescs=|t  LocalVarLogging=[]
  PWM : Scope  Commented=on
      settings: TimeRange=2  YMin=-1  YMax=6  SaveName=RPM  SampleTime=0.1
  Rv : Scope  Commented=on
      settings: TimeRange=2  YMin=-1  YMax=6  SaveName=RPM1  SampleTime=0.1
  Solver Configuration : nesl_utility/Solver Configuration  PhysicalDomain=network_engine_domain  SubClassName=solver  LeftPortType=input  RightPortType=generic  Accelerate=off  Tones=[]  Harmonics=[]  SimulateNoise=off  Profile=off  UseLocalSampling=off  EnableSwitchedLinearOptims=on  FrequencyDomain=off  UseCCode=off  UseNewInitialization=off  DoDC=off  ResidualTolerance=1e-9  UseLocalSolver=off  LocalSolverChoice=NE_BACKWARD_EULER_ADVANCER  LocalSolverSampleTime=.001  DoFixedCost=off  MaxNonlinIter=3  MaxModeIter=2  LinearAlgebra=Sparse  DelaysMemoryBudget=1024
  Stepper Controller : Subsystem  BlockChoice=Position Controller
      link override Position Controller/Control algorithm implemented on a microprocessor or dedicated discrete chip/Logic2Volts1: Gain=5
      link override Position Controller/Control algorithm implemented on a microprocessor or dedicated discrete chip/Logic2Volts2: Gain=5
      link override Position Controller/Control algorithm implemented on a microprocessor or dedicated discrete chip/Pulse Generator: f=5000
      settings: AttributesFormatString=%<BlockChoice>  MemberBlocks=Position Controller,Speed Controller
      settings: TemplateBlock=|
      | elec_controlled_stepper_lib/Configurable
      | Subsystem
  Stepper Motor : elec_lib/Actuators & Drivers/Rotational Actuators/Stepper Motor  Ra=1.04 Ohm  La=2.2 mH  Km=0.14 N*m/A  Rm=Inf Ohm  Step=1.8 deg  J=4.5e-5 kg*m^2  B=8e-4 N*m/(rad/s)  speed0=0 rpm  theta0=0 deg  LocalVarLogging=[]  alpha=[ 0.00393 0.00393 ] 1/K  Tmeas=25 C  thermal_masses=[ 100 100 ] J/K  initial_temperatures=[ 25 25 ] C  rotor_thermal_mass=50 J/K  rotor_initial_temperature=25 C  Rm_percent_rotor=90
  Stepper Motor Driver : elec_lib/Actuators & Drivers/Drivers/Stepper Motor Driver  Venable=2.5 V  Vreverse=2.5 V  Vm=24 V  LocalVarLogging=[]
  PS Torque : PMIOPort  Port=1  Side=Left
  "Dir " : Outport
  wires:
  Meas 1/1(SL) -> PWM/1
  In1/1 -> Stepper Controller/1(Ref)
  Meas 2/1(SL) -> "Dir "/1, Rv/1
  connections:
  Electrical Reference3/LConn1 -- Stepper Motor/LConn1 -- Stepper Motor Driver/RConn1
  Electrical Reference2/LConn1 -- Stepper Motor/LConn4 -- Stepper Motor Driver/RConn4
  Load Sensors/LConn1 -- Stepper Motor/RConn1 -- Solver Configuration/RConn1
  Mechanical Rotational Reference1/LConn1 -- Stepper Motor/RConn2 -- Load Sensors/LConn2
  Stepper Motor Driver/LConn1 -- Stepper Controller/RConn1 -- Meas 1/LConn1
  Stepper Controller/RConn2 -- Stepper Motor Driver/LConn2
  Stepper Motor/LConn2 -- Stepper Motor Driver/RConn2
  Stepper Motor/LConn3 -- Stepper Motor Driver/RConn3
  Stepper Controller/RConn3 -- Meas 2/LConn1 -- Stepper Motor Driver/LConn3
  Load Sensors/RConn1 -- PS Torque/RConn1

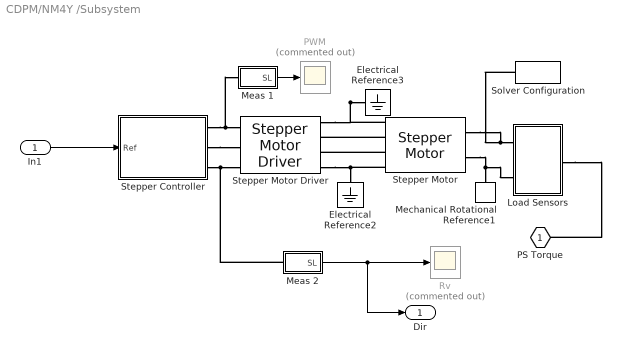
== system CDPM/NM4Y /Subsystem ==
  In1 : Inport
  Electrical Reference2 : fl_lib/Electrical/Electrical Elements/Electrical Reference  i_Log=off  LocalVarNames=|i  LocalVarDescs=|i  LocalVarLogging=[]
  Electrical Reference3 : fl_lib/Electrical/Electrical Elements/Electrical Reference  i_Log=off  LocalVarNames=|i  LocalVarDescs=|i  LocalVarLogging=[]
  Load Sensors : Subsystem
  Meas 1 : Subsystem
  Meas 2 : Subsystem
  Mechanical Rotational Reference1 : fl_lib/Mechanical/Rotational Elements/Mechanical Rotational Reference  t_Log=off  LocalVarNames=|t  LocalVarDescs=|t  LocalVarLogging=[]
  PWM : Scope  Commented=on
      settings: TimeRange=2  YMin=-1  YMax=6  SaveName=RPM  SampleTime=0.1
  Rv : Scope  Commented=on
      settings: TimeRange=2  YMin=-1  YMax=6  SaveName=RPM1  SampleTime=0.1
  Solver Configuration : nesl_utility/Solver Configuration  PhysicalDomain=network_engine_domain  SubClassName=solver  LeftPortType=input  RightPortType=generic  Accelerate=off  Tones=[]  Harmonics=[]  SimulateNoise=off  Profile=off  UseLocalSampling=off  EnableSwitchedLinearOptims=on  FrequencyDomain=off  UseCCode=off  UseNewInitialization=off  DoDC=off  ResidualTolerance=1e-9  UseLocalSolver=off  LocalSolverChoice=NE_BACKWARD_EULER_ADVANCER  LocalSolverSampleTime=.001  DoFixedCost=off  MaxNonlinIter=3  MaxModeIter=2  LinearAlgebra=Sparse  DelaysMemoryBudget=1024
  Stepper Controller : Subsystem  BlockChoice=Position Controller
      link override Position Controller/Control algorithm implemented on a microprocessor or dedicated discrete chip/Logic2Volts1: Gain=5
      link override Position Controller/Control algorithm implemented on a microprocessor or dedicated discrete chip/Logic2Volts2: Gain=5
      link override Position Controller/Control algorithm implemented on a microprocessor or dedicated discrete chip/Pulse Generator: f=5000
      settings: AttributesFormatString=%<BlockChoice>  MemberBlocks=Position Controller,Speed Controller
      settings: TemplateBlock=|
      | elec_controlled_stepper_lib/Configurable
      | Subsystem
  Stepper Motor : elec_lib/Actuators & Drivers/Rotational Actuators/Stepper Motor  Ra=1.04 Ohm  La=2.2 mH  Km=0.14 N*m/A  Rm=Inf Ohm  Step=1.8 deg  J=4.5e-5 kg*m^2  B=8e-4 N*m/(rad/s)  speed0=0 rpm  theta0=0 deg  LocalVarLogging=[]  alpha=[ 0.00393 0.00393 ] 1/K  Tmeas=25 C  thermal_masses=[ 100 100 ] J/K  initial_temperatures=[ 25 25 ] C  rotor_thermal_mass=50 J/K  rotor_initial_temperature=25 C  Rm_percent_rotor=90
  Stepper Motor Driver : elec_lib/Actuators & Drivers/Drivers/Stepper Motor Driver  Venable=2.5 V  Vreverse=2.5 V  Vm=24 V  LocalVarLogging=[]
  PS Torque : PMIOPort  Port=1  Side=Left
  "Dir " : Outport
  wires:
  Meas 1/1(SL) -> PWM/1
  In1/1 -> Stepper Controller/1(Ref)
  Meas 2/1(SL) -> "Dir "/1, Rv/1
  connections:
  Electrical Reference3/LConn1 -- Stepper Motor/LConn1 -- Stepper Motor Driver/RConn1
  Electrical Reference2/LConn1 -- Stepper Motor/LConn4 -- Stepper Motor Driver/RConn4
  Load Sensors/LConn1 -- Stepper Motor/RConn1 -- Solver Configuration/RConn1
  Mechanical Rotational Reference1/LConn1 -- Stepper Motor/RConn2 -- Load Sensors/LConn2
  Stepper Motor Driver/LConn1 -- Stepper Controller/RConn1 -- Meas 1/LConn1
  Stepper Controller/RConn2 -- Stepper Motor Driver/LConn2
  Stepper Motor/LConn2 -- Stepper Motor Driver/RConn2
  Stepper Motor/LConn3 -- Stepper Motor Driver/RConn3
  Stepper Controller/RConn3 -- Meas 2/LConn1 -- Stepper Motor Driver/LConn3
  Load Sensors/RConn1 -- PS Torque/RConn1

== system CDPM/Subsystem3/Herons Formula ==
  In1 : Inport
  In2 : Inport  Port=2
  In3 : Inport  Port=3
  Add : Sum  Inputs=+++
  Subsystem : Subsystem
  Out1 : Outport
  wires:
  In1/1 -> Subsystem/1(In1), Add/1
  In3/1 -> Subsystem/4(In4), Add/3
  In2/1 -> Subsystem/3(In3), Add/2
  Add/1 -> Subsystem/2(In2)
  Subsystem/1(Out1) -> Out1/1

== system CDPM/Subsystem3/Herons Formula1 ==
  In1 : Inport
  In2 : Inport  Port=2
  In3 : Inport  Port=3
  Add : Sum  Inputs=+++
  Subsystem : Subsystem
  Out1 : Outport
  wires:
  In1/1 -> Subsystem/1(In1), Add/1
  In3/1 -> Subsystem/4(In4), Add/3
  In2/1 -> Subsystem/3(In3), Add/2
  Add/1 -> Subsystem/2(In2)
  Subsystem/1(Out1) -> Out1/1

== system CDPM/Main Control /Subsystem/D Resolution  ==
  In1 : Inport
  Submatrix : dspmtrx3/Submatrix  RowSpan=All rows  RowStartMode=First  RowStartIndex=1  RowEndMode=Last  RowEndIndex=1  ColSpan=One column  ColStartMode=Index  ColStartIndex=1  ColEndMode=Last  ColEndIndex=1
  Submatrix1 : dspmtrx3/Submatrix  RowSpan=One row  RowStartMode=Index  RowStartIndex=1  RowEndMode=Last  RowEndIndex=1  ColSpan=One column  ColStartMode=Index  ColStartIndex=2  ColEndMode=Last  ColEndIndex=1
  Submatrix2 : dspmtrx3/Submatrix  RowSpan=All rows  RowStartMode=Index  RowStartIndex=2  RowEndMode=Last  RowEndIndex=1  ColSpan=One column  ColStartMode=Index  ColStartIndex=3  ColEndMode=Last  ColEndIndex=1
  Submatrix3 : dspmtrx3/Submatrix  RowSpan=All rows  RowStartMode=Index  RowStartIndex=2  RowEndMode=Last  RowEndIndex=1  ColSpan=One column  ColStartMode=Index  ColStartIndex=4  ColEndMode=Last  ColEndIndex=1
  Out1 : Outport
  Out2 : Outport  Port=2
  Out3 : Outport  Port=3
  Out4 : Outport  Port=4
  wires:
  Submatrix2/1 -> Out3/1
  Submatrix1/1 -> Out2/1
  Submatrix3/1 -> Out4/1
  Submatrix/1 -> Out1/1
  In1/1 -> Submatrix/1, Submatrix1/1, Submatrix2/1, Submatrix3/1

== system CDPM/Main Control /Subsystem1/D Resolution 1 ==
  In1 : Inport
  Submatrix : dspmtrx3/Submatrix  RowSpan=All rows  RowStartMode=First  RowStartIndex=1  RowEndMode=Last  RowEndIndex=1  ColSpan=One column  ColStartMode=Index  ColStartIndex=1  ColEndMode=Last  ColEndIndex=1
  Submatrix1 : dspmtrx3/Submatrix  RowSpan=One row  RowStartMode=Index  RowStartIndex=1  RowEndMode=Last  RowEndIndex=1  ColSpan=One column  ColStartMode=Index  ColStartIndex=2  ColEndMode=Last  ColEndIndex=1
  Submatrix2 : dspmtrx3/Submatrix  RowSpan=All rows  RowStartMode=Index  RowStartIndex=2  RowEndMode=Last  RowEndIndex=1  ColSpan=One column  ColStartMode=Index  ColStartIndex=3  ColEndMode=Last  ColEndIndex=1
  Submatrix3 : dspmtrx3/Submatrix  RowSpan=All rows  RowStartMode=Index  RowStartIndex=2  RowEndMode=Last  RowEndIndex=1  ColSpan=One column  ColStartMode=Index  ColStartIndex=4  ColEndMode=Last  ColEndIndex=1
  Out1 : Outport
  Out2 : Outport  Port=2
  Out3 : Outport  Port=3
  Out4 : Outport  Port=4
  wires:
  Submatrix2/1 -> Out3/1
  Submatrix1/1 -> Out2/1
  Submatrix3/1 -> Out4/1
  Submatrix/1 -> Out1/1
  In1/1 -> Submatrix/1, Submatrix1/1, Submatrix2/1, Submatrix3/1

== system CDPM/NM1R /Subsystem/Load Sensors ==
  Ideal Torque Sensor : fl_lib/Mechanical/Mechanical Sensors/Ideal Torque Sensor  w_Log=off  t_Log=off  LocalVarNames=|w|t  LocalVarDescs=|w|t  LocalVarLogging=[0 0]
  R : PMIOPort  Port=1  Side=Left
  C : PMIOPort  Port=2  Side=Left
  "Torque " : PMIOPort  Port=3  Side=Right
  connections:
  Ideal Torque Sensor/LConn1 -- R/RConn1
  Ideal Torque Sensor/RConn1 -- C/RConn1
  "Torque "/RConn1 -- Ideal Torque Sensor/RConn2

== system CDPM/NM1R /Subsystem/Meas 1 ==
  Electrical Reference : fl_lib/Electrical/Electrical Elements/Electrical Reference  i_Log=off  LocalVarNames=|i  LocalVarDescs=|i  LocalVarLogging=[]
  PS-Simulink Converter : nesl_utility/PS-Simulink Converter  PhysicalDomain=network_engine_domain  SubClassName=ps_output  LeftPortType=input  RightPortType=output  PseudoPeriodic=off  Frequencies=[]  Unit=V  AffineConversion=off
  Voltage Sensor : fl_lib/Electrical/Electrical Sensors/Voltage Sensor  i1_Log=off  v1_Log=off  LocalVarNames=|i1|v1  LocalVarDescs=|i1|v1  LocalVarLogging=[]
  V : PMIOPort  Port=1  Side=Left
  SL : Outport
  wires:
  PS-Simulink Converter/1 -> SL/1
  connections:
  V/RConn1 -- Voltage Sensor/LConn1
  Electrical Reference/LConn1 -- Voltage Sensor/RConn2
  Voltage Sensor/RConn1 -- PS-Simulink Converter/LConn1

== system CDPM/NM1R /Subsystem/Meas 2 ==
  Electrical Reference : fl_lib/Electrical/Electrical Elements/Electrical Reference  i_Log=off  LocalVarNames=|i  LocalVarDescs=|i  LocalVarLogging=[]
  PS-Simulink Converter : nesl_utility/PS-Simulink Converter  PhysicalDomain=network_engine_domain  SubClassName=ps_output  LeftPortType=input  RightPortType=output  PseudoPeriodic=off  Frequencies=[]  Unit=V  AffineConversion=off
  Voltage Sensor : fl_lib/Electrical/Electrical Sensors/Voltage Sensor  i1_Log=off  v1_Log=off  LocalVarNames=|i1|v1  LocalVarDescs=|i1|v1  LocalVarLogging=[]
  V : PMIOPort  Port=1  Side=Left
  SL : Outport
  wires:
  PS-Simulink Converter/1 -> SL/1
  connections:
  V/RConn1 -- Voltage Sensor/LConn1
  Electrical Reference/LConn1 -- Voltage Sensor/RConn2
  Voltage Sensor/RConn1 -- PS-Simulink Converter/LConn1

== system CDPM/NM1R /Subsystem/Stepper Controller ==
  Ref : Inport
  Position Controller : elec_controlled_stepper_lib/Position Controller
  PWM : PMIOPort  Port=1  Side=Right
  0v : PMIOPort  Port=2  Side=Right
  REV : PMIOPort  Port=3  Side=Right
  wires:
  Ref/1 -> Position Controller/1
  connections:
  Position Controller/RConn1 -- PWM/RConn1
  Position Controller/RConn2 -- 0v/RConn1
  Position Controller/RConn3 -- REV/RConn1

== system CDPM/NM2B/Subsystem/Load Sensors ==
  Ideal Torque Sensor : fl_lib/Mechanical/Mechanical Sensors/Ideal Torque Sensor  w_Log=off  t_Log=off  LocalVarNames=|w|t  LocalVarDescs=|w|t  LocalVarLogging=[0 0]
  R : PMIOPort  Port=1  Side=Left
  C : PMIOPort  Port=2  Side=Left
  "Torque " : PMIOPort  Port=3  Side=Right
  connections:
  Ideal Torque Sensor/LConn1 -- R/RConn1
  Ideal Torque Sensor/RConn1 -- C/RConn1
  "Torque "/RConn1 -- Ideal Torque Sensor/RConn2

== system CDPM/NM2B/Subsystem/Meas 1 ==
  Electrical Reference : fl_lib/Electrical/Electrical Elements/Electrical Reference  i_Log=off  LocalVarNames=|i  LocalVarDescs=|i  LocalVarLogging=[]
  PS-Simulink Converter : nesl_utility/PS-Simulink Converter  PhysicalDomain=network_engine_domain  SubClassName=ps_output  LeftPortType=input  RightPortType=output  PseudoPeriodic=off  Frequencies=[]  Unit=V  AffineConversion=off
  Voltage Sensor : fl_lib/Electrical/Electrical Sensors/Voltage Sensor  i1_Log=off  v1_Log=off  LocalVarNames=|i1|v1  LocalVarDescs=|i1|v1  LocalVarLogging=[]
  V : PMIOPort  Port=1  Side=Left
  SL : Outport
  wires:
  PS-Simulink Converter/1 -> SL/1
  connections:
  V/RConn1 -- Voltage Sensor/LConn1
  Electrical Reference/LConn1 -- Voltage Sensor/RConn2
  Voltage Sensor/RConn1 -- PS-Simulink Converter/LConn1

== system CDPM/NM2B/Subsystem/Meas 2 ==
  Electrical Reference : fl_lib/Electrical/Electrical Elements/Electrical Reference  i_Log=off  LocalVarNames=|i  LocalVarDescs=|i  LocalVarLogging=[]
  PS-Simulink Converter : nesl_utility/PS-Simulink Converter  PhysicalDomain=network_engine_domain  SubClassName=ps_output  LeftPortType=input  RightPortType=output  PseudoPeriodic=off  Frequencies=[]  Unit=V  AffineConversion=off
  Voltage Sensor : fl_lib/Electrical/Electrical Sensors/Voltage Sensor  i1_Log=off  v1_Log=off  LocalVarNames=|i1|v1  LocalVarDescs=|i1|v1  LocalVarLogging=[]
  V : PMIOPort  Port=1  Side=Left
  SL : Outport
  wires:
  PS-Simulink Converter/1 -> SL/1
  connections:
  V/RConn1 -- Voltage Sensor/LConn1
  Electrical Reference/LConn1 -- Voltage Sensor/RConn2
  Voltage Sensor/RConn1 -- PS-Simulink Converter/LConn1

== system CDPM/NM2B/Subsystem/Stepper Controller ==
  Ref : Inport
  Position Controller : elec_controlled_stepper_lib/Position Controller
  PWM : PMIOPort  Port=1  Side=Right
  0v : PMIOPort  Port=2  Side=Right
  REV : PMIOPort  Port=3  Side=Right
  wires:
  Ref/1 -> Position Controller/1
  connections:
  Position Controller/RConn1 -- PWM/RConn1
  Position Controller/RConn2 -- 0v/RConn1
  Position Controller/RConn3 -- REV/RConn1

== system CDPM/NM3G/Subsystem/Load Sensors ==
  Ideal Torque Sensor : fl_lib/Mechanical/Mechanical Sensors/Ideal Torque Sensor  w_Log=off  t_Log=off  LocalVarNames=|w|t  LocalVarDescs=|w|t  LocalVarLogging=[0 0]
  R : PMIOPort  Port=1  Side=Left
  C : PMIOPort  Port=2  Side=Left
  "Torque " : PMIOPort  Port=3  Side=Right
  connections:
  Ideal Torque Sensor/LConn1 -- R/RConn1
  Ideal Torque Sensor/RConn1 -- C/RConn1
  "Torque "/RConn1 -- Ideal Torque Sensor/RConn2

== system CDPM/NM3G/Subsystem/Meas 1 ==
  Electrical Reference : fl_lib/Electrical/Electrical Elements/Electrical Reference  i_Log=off  LocalVarNames=|i  LocalVarDescs=|i  LocalVarLogging=[]
  PS-Simulink Converter : nesl_utility/PS-Simulink Converter  PhysicalDomain=network_engine_domain  SubClassName=ps_output  LeftPortType=input  RightPortType=output  PseudoPeriodic=off  Frequencies=[]  Unit=V  AffineConversion=off
  Voltage Sensor : fl_lib/Electrical/Electrical Sensors/Voltage Sensor  i1_Log=off  v1_Log=off  LocalVarNames=|i1|v1  LocalVarDescs=|i1|v1  LocalVarLogging=[]
  V : PMIOPort  Port=1  Side=Left
  SL : Outport
  wires:
  PS-Simulink Converter/1 -> SL/1
  connections:
  V/RConn1 -- Voltage Sensor/LConn1
  Electrical Reference/LConn1 -- Voltage Sensor/RConn2
  Voltage Sensor/RConn1 -- PS-Simulink Converter/LConn1

== system CDPM/NM3G/Subsystem/Meas 2 ==
  Electrical Reference : fl_lib/Electrical/Electrical Elements/Electrical Reference  i_Log=off  LocalVarNames=|i  LocalVarDescs=|i  LocalVarLogging=[]
  PS-Simulink Converter : nesl_utility/PS-Simulink Converter  PhysicalDomain=network_engine_domain  SubClassName=ps_output  LeftPortType=input  RightPortType=output  PseudoPeriodic=off  Frequencies=[]  Unit=V  AffineConversion=off
  Voltage Sensor : fl_lib/Electrical/Electrical Sensors/Voltage Sensor  i1_Log=off  v1_Log=off  LocalVarNames=|i1|v1  LocalVarDescs=|i1|v1  LocalVarLogging=[]
  V : PMIOPort  Port=1  Side=Left
  SL : Outport
  wires:
  PS-Simulink Converter/1 -> SL/1
  connections:
  V/RConn1 -- Voltage Sensor/LConn1
  Electrical Reference/LConn1 -- Voltage Sensor/RConn2
  Voltage Sensor/RConn1 -- PS-Simulink Converter/LConn1

== system CDPM/NM3G/Subsystem/Stepper Controller ==
  Ref : Inport
  Position Controller : elec_controlled_stepper_lib/Position Controller
  PWM : PMIOPort  Port=1  Side=Right
  0v : PMIOPort  Port=2  Side=Right
  REV : PMIOPort  Port=3  Side=Right
  wires:
  Ref/1 -> Position Controller/1
  connections:
  Position Controller/RConn1 -- PWM/RConn1
  Position Controller/RConn2 -- 0v/RConn1
  Position Controller/RConn3 -- REV/RConn1

== system CDPM/NM4Y /Subsystem/Load Sensors ==
  Ideal Torque Sensor : fl_lib/Mechanical/Mechanical Sensors/Ideal Torque Sensor  w_Log=off  t_Log=off  LocalVarNames=|w|t  LocalVarDescs=|w|t  LocalVarLogging=[0 0]
  R : PMIOPort  Port=1  Side=Left
  C : PMIOPort  Port=2  Side=Left
  "Torque " : PMIOPort  Port=3  Side=Right
  connections:
  Ideal Torque Sensor/LConn1 -- R/RConn1
  Ideal Torque Sensor/RConn1 -- C/RConn1
  "Torque "/RConn1 -- Ideal Torque Sensor/RConn2
